simulink subsystem "tcp_trace_simscape_ref_subsys"  (R2022b)
settings: Solver=VariableStepAuto  StartTime=0.0  StopTime=10.0  RelTol=1e-3
undefined symbols (not defined in the file): param_vis
libraries: nesl_utility x300, sm_lib x200
(part 3 of 3)

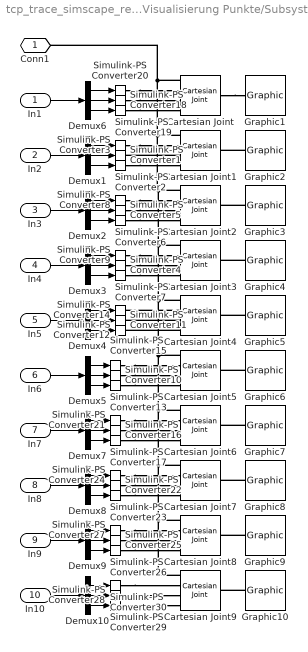
== system tcp_trace_simscape_ref_subsys/Visualisierung Punkte/Subsystem8 ==
  In1 : Inport
  In2 : Inport  Port=2
  In3 : Inport  Port=3
  In4 : Inport  Port=4
  In5 : Inport  Port=5
  In6 : Inport  Port=6
  In7 : Inport  Port=7
  In8 : Inport  Port=8
  In9 : Inport  Port=9
  In10 : Inport  Port=10
  Cartesian Joint{,1..9} (10 alike) : sm_lib/Joints/Cartesian Joint  JointMode=Normal  SenseConstraintForce=off  SenseConstraintForceX=off  SenseConstraintForceY=off  SenseConstraintForceZ=off  SenseConstraintTorque=off  SenseConstraintTorqueX=off  SenseConstraintTorqueY=off  SenseConstraintTorqueZ=off  SenseTotalForce=off  SenseTotalForceX=off  SenseTotalForceY=off  SenseTotalForceZ=off  SenseTotalTorque=off  SenseTotalTorqueX=off  SenseTotalTorqueY=off  SenseTotalTorqueZ=off  CompositeWrenchDir=FollowerOnBase  CompositeWrenchFrame=BaseFrame  PxEquilibriumPosition=0  PxEquilibriumPositionUnits=m  PxSpringStiffness=0  PxSpringStiffnessUnits=N/m  PxDampingCoefficient=0  PxDampingCoefficientUnits=N/(m/s)  PxTorqueActuationMode=ComputedTorque  PxMotionActuationMode=InputMotion  PxSensePosition=off  PxSenseVelocity=off  PxSenseAcceleration=off  PxSenseTorqueForce=off  PxSenseLowerLimitTorqueForce=off  PxSenseUpperLimitTorqueForce=off  PxLowerLimitSpecify=off  PxLowerLimitBound=-1  PxLowerLimitBoundUnits=m  PxLowerLimitStiffness=1e6  PxLowerLimitStiffnessUnits=N/m  PxLowerLimitDamping=1e3  PxLowerLimitDampingUnits=N/(m/s)  PxLowerLimitTransitionRegionWidth=1e-4  PxLowerLimitTransitionRegionWidthUnits=m  PxUpperLimitSpecify=off  PxUpperLimitBound=1  PxUpperLimitBoundUnits=m  PxUpperLimitStiffness=1e6  PxUpperLimitStiffnessUnits=N/m  PxUpperLimitDamping=1e3  PxUpperLimitDampingUnits=N/(m/s)  PxUpperLimitTransitionRegionWidth=1e-4  PxUpperLimitTransitionRegionWidthUnits=m  PxPositionTargetSpecify=off  PxPositionTargetPriority=High  PxPositionTargetValue=0  PxPositionTargetValueUnits=m  PxVelocityTargetSpecify=off  PxVelocityTargetPriority=High  PxVelocityTargetValue=0  PxVelocityTargetValueUnits=m/s  PyEquilibriumPosition=0  PyEquilibriumPositionUnits=m  PySpringStiffness=0  PySpringStiffnessUnits=N/m  PyDampingCoefficient=0  PyDampingCoefficientUnits=N/(m/s)  PyTorqueActuationMode=ComputedTorque  PyMotionActuationMode=InputMotion  PySensePosition=off  PySenseVelocity=off  PySenseAcceleration=off  PySenseTorqueForce=off  PySenseLowerLimitTorqueForce=off  PySenseUpperLimitTorqueForce=off  PyLowerLimitSpecify=off  PyLowerLimitBound=-1  PyLowerLimitBoundUnits=m  PyLowerLimitStiffness=1e6  PyLowerLimitStiffnessUnits=N/m  PyLowerLimitDamping=1e3  PyLowerLimitDampingUnits=N/(m/s)  PyLowerLimitTransitionRegionWidth=1e-4  PyLowerLimitTransitionRegionWidthUnits=m  PyUpperLimitSpecify=off  PyUpperLimitBound=1  PyUpperLimitBoundUnits=m  PyUpperLimitStiffness=1e6  PyUpperLimitStiffnessUnits=N/m  PyUpperLimitDamping=1e3  PyUpperLimitDampingUnits=N/(m/s)  PyUpperLimitTransitionRegionWidth=1e-4  PyUpperLimitTransitionRegionWidthUnits=m  PyPositionTargetSpecify=off  PyPositionTargetPriority=High  PyPositionTargetValue=0  PyPositionTargetValueUnits=m  PyVelocityTargetSpecify=off  PyVelocityTargetPriority=High  PyVelocityTargetValue=0  PyVelocityTargetValueUnits=m/s  PzEquilibriumPosition=0  PzEquilibriumPositionUnits=m  PzSpringStiffness=0  PzSpringStiffnessUnits=N/m  PzDampingCoefficient=0  PzDampingCoefficientUnits=N/(m/s)  PzTorqueActuationMode=ComputedTorque  PzMotionActuationMode=InputMotion  PzSensePosition=off  PzSenseVelocity=off  PzSenseAcceleration=off  PzSenseTorqueForce=off  PzSenseLowerLimitTorqueForce=off  PzSenseUpperLimitTorqueForce=off  PzLowerLimitSpecify=off  PzLowerLimitBound=-1  PzLowerLimitBoundUnits=m  PzLowerLimitStiffness=1e6  PzLowerLimitStiffnessUnits=N/m  PzLowerLimitDamping=1e3  PzLowerLimitDampingUnits=N/(m/s)  PzLowerLimitTransitionRegionWidth=1e-4  PzLowerLimitTransitionRegionWidthUnits=m  PzUpperLimitSpecify=off  PzUpperLimitBound=1  PzUpperLimitBoundUnits=m  PzUpperLimitStiffness=1e6  PzUpperLimitStiffnessUnits=N/m  PzUpperLimitDamping=1e3  PzUpperLimitDampingUnits=N/(m/s)  PzUpperLimitTransitionRegionWidth=1e-4  PzUpperLimitTransitionRegionWidthUnits=m  PzPositionTargetSpecify=off  PzPositionTargetPriority=High  PzPositionTargetValue=0  PzPositionTargetValueUnits=m  PzVelocityTargetSpecify=off  PzVelocityTargetPriority=High  PzVelocityTargetValue=0  PzVelocityTargetValueUnits=m/s
  Demux{1..10} (10 alike) : Demux  Outputs=3
  Graphic{1..10} (10 alike) : sm_lib/Body Elements/Graphic  GraphicType=Marker  MarkerShape=Sphere  MarkerSize=param_vis.vis_point.pix  GraphicVisPropType=SimpleVisualProperties  GraphicDiffuseColor=param_vis.vis_point.col  GraphicSpecularColor=[0.5 0.5 0.5 1.0]  GraphicAmbientColor=[0.15 0.15 0.15 1.0]  GraphicEmissiveColor=[0.0 0.0 0.0 1.0]  GraphicShininess=75  GraphicOpacity=param_vis.vis_point.opa
  Simulink-PS Converter{1..30} (30 alike) : nesl_utility/Simulink-PS Converter  PhysicalDomain=network_engine_domain  SubClassName=ps_input  LeftPortType=input  RightPortType=output  PseudoPeriodic=off  Frequencies=[]  NoiseDistribution=none  NoiseParameters=[]  Unit=1  AffineConversion=off  FilteringAndDerivatives=zero  SimscapeFilterOrder=2  InputFilterTimeConstant=0.001  UdotUserProvided=0
  Conn1 : PMIOPort  Side=Left
  wires:
  In7/1 -> Demux7/1
  In6/1 -> Demux5/1
  In10/1 -> Demux10/1
  In2/1 -> Demux1/1
  In5/1 -> Demux4/1
  In4/1 -> Demux3/1
  Demux6/3 -> Simulink-PS Converter19/1
  In3/1 -> Demux2/1
  In1/1 -> Demux6/1
  In9/1 -> Demux9/1
  In8/1 -> Demux8/1
  Demux6/1 -> Simulink-PS Converter20/1
  Demux6/2 -> Simulink-PS Converter18/1
  Demux1/1 -> Simulink-PS Converter3/1
  Demux4/2 -> Simulink-PS Converter11/1
  Demux4/1 -> Simulink-PS Converter14/1
  Demux4/3 -> Simulink-PS Converter12/1
  Demux1/2 -> Simulink-PS Converter1/1
  Demux1/3 -> Simulink-PS Converter2/1
  Demux2/1 -> Simulink-PS Converter8/1
  Demux2/2 -> Simulink-PS Converter5/1
  Demux2/3 -> Simulink-PS Converter6/1
  Demux3/3 -> Simulink-PS Converter7/1
  Demux3/1 -> Simulink-PS Converter9/1
  Demux3/2 -> Simulink-PS Converter4/1
  Demux5/1 -> Simulink-PS Converter15/1
  Demux5/2 -> Simulink-PS Converter10/1
  Demux5/3 -> Simulink-PS Converter13/1
  Demux7/1 -> Simulink-PS Converter21/1
  Demux7/2 -> Simulink-PS Converter16/1
  Demux7/3 -> Simulink-PS Converter17/1
  Demux8/1 -> Simulink-PS Converter24/1
  Demux8/2 -> Simulink-PS Converter22/1
  Demux8/3 -> Simulink-PS Converter23/1
  Demux9/1 -> Simulink-PS Converter27/1
  Demux9/2 -> Simulink-PS Converter25/1
  Demux9/3 -> Simulink-PS Converter26/1
  Demux10/1 -> Simulink-PS Converter30/1
  Demux10/2 -> Simulink-PS Converter28/1
  Demux10/3 -> Simulink-PS Converter29/1
  connections:
  Simulink-PS Converter19/RConn1 -- Cartesian Joint/LConn4
  Graphic4/RConn1 -- Cartesian Joint3/RConn1
  Cartesian Joint/RConn1 -- Graphic1/RConn1
  Graphic3/RConn1 -- Cartesian Joint2/RConn1
  Cartesian Joint8/LConn1 -- Cartesian Joint9/LConn1 -- Cartesian Joint7/LConn1 -- Cartesian Joint6/LConn1 -- Cartesian Joint5/LConn1 -- Cartesian Joint4/LConn1 -- Cartesian Joint3/LConn1 -- Cartesian Joint2/LConn1 -- Cartesian Joint1/LConn1 -- Cartesian Joint/LConn1 -- Conn1/RConn1
  Graphic7/RConn1 -- Cartesian Joint6/RConn1
  Graphic8/RConn1 -- Cartesian Joint7/RConn1
  Graphic6/RConn1 -- Cartesian Joint5/RConn1
  Graphic9/RConn1 -- Cartesian Joint8/RConn1
  Graphic2/RConn1 -- Cartesian Joint1/RConn1
  Graphic5/RConn1 -- Cartesian Joint4/RConn1
  Graphic10/RConn1 -- Cartesian Joint9/RConn1
  Simulink-PS Converter18/RConn1 -- Cartesian Joint/LConn3
  Simulink-PS Converter20/RConn1 -- Cartesian Joint/LConn2
  Simulink-PS Converter6/RConn1 -- Cartesian Joint2/LConn4
  Simulink-PS Converter8/RConn1 -- Cartesian Joint2/LConn2
  Simulink-PS Converter5/RConn1 -- Cartesian Joint2/LConn3
  Cartesian Joint4/LConn4 -- Simulink-PS Converter12/RConn1
  Cartesian Joint4/LConn2 -- Simulink-PS Converter14/RConn1
  Cartesian Joint4/LConn3 -- Simulink-PS Converter11/RConn1
  Simulink-PS Converter3/RConn1 -- Cartesian Joint1/LConn2
  Cartesian Joint1/LConn3 -- Simulink-PS Converter1/RConn1
  Simulink-PS Converter2/RConn1 -- Cartesian Joint1/LConn4
  Simulink-PS Converter15/RConn1 -- Cartesian Joint5/LConn2
  Simulink-PS Converter10/RConn1 -- Cartesian Joint5/LConn3
  Simulink-PS Converter13/RConn1 -- Cartesian Joint5/LConn4
  Simulink-PS Converter21/RConn1 -- Cartesian Joint6/LConn2
  Simulink-PS Converter16/RConn1 -- Cartesian Joint6/LConn3
  Simulink-PS Converter17/RConn1 -- Cartesian Joint6/LConn4
  Simulink-PS Converter24/RConn1 -- Cartesian Joint7/LConn2
  Simulink-PS Converter22/RConn1 -- Cartesian Joint7/LConn3
  Simulink-PS Converter23/RConn1 -- Cartesian Joint7/LConn4
  Simulink-PS Converter27/RConn1 -- Cartesian Joint8/LConn2
  Simulink-PS Converter25/RConn1 -- Cartesian Joint8/LConn3
  Simulink-PS Converter26/RConn1 -- Cartesian Joint8/LConn4
  Simulink-PS Converter30/RConn1 -- Cartesian Joint9/LConn2
  Simulink-PS Converter28/RConn1 -- Cartesian Joint9/LConn3
  Simulink-PS Converter29/RConn1 -- Cartesian Joint9/LConn4
  Simulink-PS Converter9/RConn1 -- Cartesian Joint3/LConn2
  Simulink-PS Converter4/RConn1 -- Cartesian Joint3/LConn3
  Simulink-PS Converter7/RConn1 -- Cartesian Joint3/LConn4

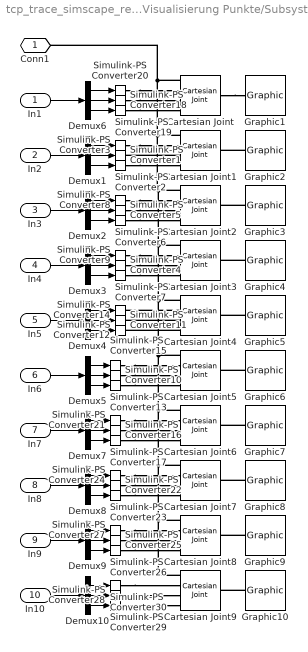
== system tcp_trace_simscape_ref_subsys/Visualisierung Punkte/Subsystem9 ==
  In1 : Inport
  In2 : Inport  Port=2
  In3 : Inport  Port=3
  In4 : Inport  Port=4
  In5 : Inport  Port=5
  In6 : Inport  Port=6
  In7 : Inport  Port=7
  In8 : Inport  Port=8
  In9 : Inport  Port=9
  In10 : Inport  Port=10
  Cartesian Joint{,1..9} (10 alike) : sm_lib/Joints/Cartesian Joint  JointMode=Normal  SenseConstraintForce=off  SenseConstraintForceX=off  SenseConstraintForceY=off  SenseConstraintForceZ=off  SenseConstraintTorque=off  SenseConstraintTorqueX=off  SenseConstraintTorqueY=off  SenseConstraintTorqueZ=off  SenseTotalForce=off  SenseTotalForceX=off  SenseTotalForceY=off  SenseTotalForceZ=off  SenseTotalTorque=off  SenseTotalTorqueX=off  SenseTotalTorqueY=off  SenseTotalTorqueZ=off  CompositeWrenchDir=FollowerOnBase  CompositeWrenchFrame=BaseFrame  PxEquilibriumPosition=0  PxEquilibriumPositionUnits=m  PxSpringStiffness=0  PxSpringStiffnessUnits=N/m  PxDampingCoefficient=0  PxDampingCoefficientUnits=N/(m/s)  PxTorqueActuationMode=ComputedTorque  PxMotionActuationMode=InputMotion  PxSensePosition=off  PxSenseVelocity=off  PxSenseAcceleration=off  PxSenseTorqueForce=off  PxSenseLowerLimitTorqueForce=off  PxSenseUpperLimitTorqueForce=off  PxLowerLimitSpecify=off  PxLowerLimitBound=-1  PxLowerLimitBoundUnits=m  PxLowerLimitStiffness=1e6  PxLowerLimitStiffnessUnits=N/m  PxLowerLimitDamping=1e3  PxLowerLimitDampingUnits=N/(m/s)  PxLowerLimitTransitionRegionWidth=1e-4  PxLowerLimitTransitionRegionWidthUnits=m  PxUpperLimitSpecify=off  PxUpperLimitBound=1  PxUpperLimitBoundUnits=m  PxUpperLimitStiffness=1e6  PxUpperLimitStiffnessUnits=N/m  PxUpperLimitDamping=1e3  PxUpperLimitDampingUnits=N/(m/s)  PxUpperLimitTransitionRegionWidth=1e-4  PxUpperLimitTransitionRegionWidthUnits=m  PxPositionTargetSpecify=off  PxPositionTargetPriority=High  PxPositionTargetValue=0  PxPositionTargetValueUnits=m  PxVelocityTargetSpecify=off  PxVelocityTargetPriority=High  PxVelocityTargetValue=0  PxVelocityTargetValueUnits=m/s  PyEquilibriumPosition=0  PyEquilibriumPositionUnits=m  PySpringStiffness=0  PySpringStiffnessUnits=N/m  PyDampingCoefficient=0  PyDampingCoefficientUnits=N/(m/s)  PyTorqueActuationMode=ComputedTorque  PyMotionActuationMode=InputMotion  PySensePosition=off  PySenseVelocity=off  PySenseAcceleration=off  PySenseTorqueForce=off  PySenseLowerLimitTorqueForce=off  PySenseUpperLimitTorqueForce=off  PyLowerLimitSpecify=off  PyLowerLimitBound=-1  PyLowerLimitBoundUnits=m  PyLowerLimitStiffness=1e6  PyLowerLimitStiffnessUnits=N/m  PyLowerLimitDamping=1e3  PyLowerLimitDampingUnits=N/(m/s)  PyLowerLimitTransitionRegionWidth=1e-4  PyLowerLimitTransitionRegionWidthUnits=m  PyUpperLimitSpecify=off  PyUpperLimitBound=1  PyUpperLimitBoundUnits=m  PyUpperLimitStiffness=1e6  PyUpperLimitStiffnessUnits=N/m  PyUpperLimitDamping=1e3  PyUpperLimitDampingUnits=N/(m/s)  PyUpperLimitTransitionRegionWidth=1e-4  PyUpperLimitTransitionRegionWidthUnits=m  PyPositionTargetSpecify=off  PyPositionTargetPriority=High  PyPositionTargetValue=0  PyPositionTargetValueUnits=m  PyVelocityTargetSpecify=off  PyVelocityTargetPriority=High  PyVelocityTargetValue=0  PyVelocityTargetValueUnits=m/s  PzEquilibriumPosition=0  PzEquilibriumPositionUnits=m  PzSpringStiffness=0  PzSpringStiffnessUnits=N/m  PzDampingCoefficient=0  PzDampingCoefficientUnits=N/(m/s)  PzTorqueActuationMode=ComputedTorque  PzMotionActuationMode=InputMotion  PzSensePosition=off  PzSenseVelocity=off  PzSenseAcceleration=off  PzSenseTorqueForce=off  PzSenseLowerLimitTorqueForce=off  PzSenseUpperLimitTorqueForce=off  PzLowerLimitSpecify=off  PzLowerLimitBound=-1  PzLowerLimitBoundUnits=m  PzLowerLimitStiffness=1e6  PzLowerLimitStiffnessUnits=N/m  PzLowerLimitDamping=1e3  PzLowerLimitDampingUnits=N/(m/s)  PzLowerLimitTransitionRegionWidth=1e-4  PzLowerLimitTransitionRegionWidthUnits=m  PzUpperLimitSpecify=off  PzUpperLimitBound=1  PzUpperLimitBoundUnits=m  PzUpperLimitStiffness=1e6  PzUpperLimitStiffnessUnits=N/m  PzUpperLimitDamping=1e3  PzUpperLimitDampingUnits=N/(m/s)  PzUpperLimitTransitionRegionWidth=1e-4  PzUpperLimitTransitionRegionWidthUnits=m  PzPositionTargetSpecify=off  PzPositionTargetPriority=High  PzPositionTargetValue=0  PzPositionTargetValueUnits=m  PzVelocityTargetSpecify=off  PzVelocityTargetPriority=High  PzVelocityTargetValue=0  PzVelocityTargetValueUnits=m/s
  Demux{1..10} (10 alike) : Demux  Outputs=3
  Graphic{1..10} (10 alike) : sm_lib/Body Elements/Graphic  GraphicType=Marker  MarkerShape=Sphere  MarkerSize=param_vis.vis_point.pix  GraphicVisPropType=SimpleVisualProperties  GraphicDiffuseColor=param_vis.vis_point.col  GraphicSpecularColor=[0.5 0.5 0.5 1.0]  GraphicAmbientColor=[0.15 0.15 0.15 1.0]  GraphicEmissiveColor=[0.0 0.0 0.0 1.0]  GraphicShininess=75  GraphicOpacity=param_vis.vis_point.opa
  Simulink-PS Converter{1..30} (30 alike) : nesl_utility/Simulink-PS Converter  PhysicalDomain=network_engine_domain  SubClassName=ps_input  LeftPortType=input  RightPortType=output  PseudoPeriodic=off  Frequencies=[]  NoiseDistribution=none  NoiseParameters=[]  Unit=1  AffineConversion=off  FilteringAndDerivatives=zero  SimscapeFilterOrder=2  InputFilterTimeConstant=0.001  UdotUserProvided=0
  Conn1 : PMIOPort  Side=Left
  wires:
  Demux10/3 -> Simulink-PS Converter29/1
  Demux10/2 -> Simulink-PS Converter28/1
  Demux10/1 -> Simulink-PS Converter30/1
  Demux9/3 -> Simulink-PS Converter26/1
  Demux9/2 -> Simulink-PS Converter25/1
  Demux9/1 -> Simulink-PS Converter27/1
  Demux8/3 -> Simulink-PS Converter23/1
  Demux8/2 -> Simulink-PS Converter22/1
  Demux8/1 -> Simulink-PS Converter24/1
  Demux7/3 -> Simulink-PS Converter17/1
  Demux7/2 -> Simulink-PS Converter16/1
  Demux7/1 -> Simulink-PS Converter21/1
  Demux5/3 -> Simulink-PS Converter13/1
  Demux5/2 -> Simulink-PS Converter10/1
  Demux5/1 -> Simulink-PS Converter15/1
  Demux3/2 -> Simulink-PS Converter4/1
  Demux3/1 -> Simulink-PS Converter9/1
  Demux3/3 -> Simulink-PS Converter7/1
  Demux2/3 -> Simulink-PS Converter6/1
  Demux2/2 -> Simulink-PS Converter5/1
  Demux2/1 -> Simulink-PS Converter8/1
  Demux1/3 -> Simulink-PS Converter2/1
  Demux1/2 -> Simulink-PS Converter1/1
  Demux4/3 -> Simulink-PS Converter12/1
  Demux4/1 -> Simulink-PS Converter14/1
  Demux4/2 -> Simulink-PS Converter11/1
  Demux1/1 -> Simulink-PS Converter3/1
  Demux6/2 -> Simulink-PS Converter18/1
  Demux6/1 -> Simulink-PS Converter20/1
  In8/1 -> Demux8/1
  In9/1 -> Demux9/1
  In1/1 -> Demux6/1
  In3/1 -> Demux2/1
  Demux6/3 -> Simulink-PS Converter19/1
  In4/1 -> Demux3/1
  In5/1 -> Demux4/1
  In2/1 -> Demux1/1
  In10/1 -> Demux10/1
  In6/1 -> Demux5/1
  In7/1 -> Demux7/1
  connections:
  Simulink-PS Converter7/RConn1 -- Cartesian Joint3/LConn4
  Simulink-PS Converter4/RConn1 -- Cartesian Joint3/LConn3
  Simulink-PS Converter9/RConn1 -- Cartesian Joint3/LConn2
  Simulink-PS Converter29/RConn1 -- Cartesian Joint9/LConn4
  Simulink-PS Converter28/RConn1 -- Cartesian Joint9/LConn3
  Simulink-PS Converter30/RConn1 -- Cartesian Joint9/LConn2
  Simulink-PS Converter26/RConn1 -- Cartesian Joint8/LConn4
  Simulink-PS Converter25/RConn1 -- Cartesian Joint8/LConn3
  Simulink-PS Converter27/RConn1 -- Cartesian Joint8/LConn2
  Simulink-PS Converter23/RConn1 -- Cartesian Joint7/LConn4
  Simulink-PS Converter22/RConn1 -- Cartesian Joint7/LConn3
  Simulink-PS Converter24/RConn1 -- Cartesian Joint7/LConn2
  Simulink-PS Converter17/RConn1 -- Cartesian Joint6/LConn4
  Simulink-PS Converter16/RConn1 -- Cartesian Joint6/LConn3
  Simulink-PS Converter21/RConn1 -- Cartesian Joint6/LConn2
  Simulink-PS Converter13/RConn1 -- Cartesian Joint5/LConn4
  Simulink-PS Converter10/RConn1 -- Cartesian Joint5/LConn3
  Simulink-PS Converter15/RConn1 -- Cartesian Joint5/LConn2
  Simulink-PS Converter2/RConn1 -- Cartesian Joint1/LConn4
  Cartesian Joint1/LConn3 -- Simulink-PS Converter1/RConn1
  Simulink-PS Converter3/RConn1 -- Cartesian Joint1/LConn2
  Cartesian Joint4/LConn3 -- Simulink-PS Converter11/RConn1
  Cartesian Joint4/LConn2 -- Simulink-PS Converter14/RConn1
  Cartesian Joint4/LConn4 -- Simulink-PS Converter12/RConn1
  Simulink-PS Converter5/RConn1 -- Cartesian Joint2/LConn3
  Simulink-PS Converter8/RConn1 -- Cartesian Joint2/LConn2
  Simulink-PS Converter6/RConn1 -- Cartesian Joint2/LConn4
  Simulink-PS Converter20/RConn1 -- Cartesian Joint/LConn2
  Simulink-PS Converter18/RConn1 -- Cartesian Joint/LConn3
  Graphic10/RConn1 -- Cartesian Joint9/RConn1
  Graphic5/RConn1 -- Cartesian Joint4/RConn1
  Graphic2/RConn1 -- Cartesian Joint1/RConn1
  Graphic9/RConn1 -- Cartesian Joint8/RConn1
  Graphic6/RConn1 -- Cartesian Joint5/RConn1
  Graphic8/RConn1 -- Cartesian Joint7/RConn1
  Graphic7/RConn1 -- Cartesian Joint6/RConn1
  Conn1/RConn1 -- Cartesian Joint/LConn1 -- Cartesian Joint1/LConn1 -- Cartesian Joint2/LConn1 -- Cartesian Joint3/LConn1 -- Cartesian Joint4/LConn1 -- Cartesian Joint5/LConn1 -- Cartesian Joint6/LConn1 -- Cartesian Joint7/LConn1 -- Cartesian Joint9/LConn1 -- Cartesian Joint8/LConn1
  Graphic3/RConn1 -- Cartesian Joint2/RConn1
  Cartesian Joint/RConn1 -- Graphic1/RConn1
  Graphic4/RConn1 -- Cartesian Joint3/RConn1
  Simulink-PS Converter19/RConn1 -- Cartesian Joint/LConn4

== matlab function tcp_trace_simscape_ref_subsys/MATLAB Function ==
  settings: updateMethod=DISCRETE  sampleTime=param_global.Ta
  data: robot_model input; p1 output; p2 output; p3 output; p4 output; p5 output; p6 output; p7 output; p8 output; p9 output; p10 output; p11 output; p12 output; p13 output; p14 output; p15 output; p16 output; p17 output; p18 output; p19 output; p20 output; p21 output; p22 output; p23 output; p24 output; p25 output; p26 output; p27 output; p28 output; p29 output; p30 output; p31 output; p32 output; p33 output; p34 output; p35 output; p36 output; p37 output; p38 output; p39 output; p40 output; p41 output; p42 output; p43 output; p44 output; p45 output; p46 output; p47 output; p48 output; p49 output; p50 output; start input; delta input; p51 output; p52 output; p53 output; p54 output; p55 output; p56 output; p57 output; p58 output; p59 output; p60 output; p61 output; p62 output; p63 output; p64 output; p65 output; p66 output; p67 output; p68 output; p69 output; p70 output; p71 output; p72 output; p73 output; p74 output; p75 output; p76 output; p77 output; p78 output; p79 output; p80 output; p81 output; p82 output; p83 output; p84 output; p85 output; p86 output; p87 output; p88 output; p89 output; p90 output; p91 output; p92 output; p93 output; p94 output; p95 output; p96 output; p97 output; p98 output; p99 output; p100 output
function [p1,p2,p3,p4,p5,p6,p7,p8,p9,p10,p11,p12,p13,p14,p15,p16,p17,p18,p19,p20,p21,p22,p23,p24,p25,p26,p27,p28,p29,p30,p31,p32,p33,p34,p35,p36,p37,p38,p39,p40,p41,p42,p43,p44,p45,p46,p47,p48,p49,p50,p51,p52,p53,p54,p55,p56,p57,p58,p59,p60,p61,p62,p63,p64,p65,p66,p67,p68,p69,p70,p71,p72,p73,p74,p75,p76,p77,p78,p79,p80,p81,p82,p83,p84,p85,p86,p87,p88,p89,p90,p91,p92,p93,p94,p95,p96,p97,p98,p99,p100] = fcn(robot_model, start, delta)
persistent i t1 t2 t3 t4 t5 t6 t7 t8 t9 t10 t11 t12 t13 t14 t15 t16 t17 t18 t19 t20 t21 t22 t23 t24 t25 t26 t27 t28 t29 t30 t31 t32 t33 t34 t35 t36 t37 t38 t39 t40 t41 t42 t43 t44 t45 t46 t47 t48 t49 t50 t51 t52 t53 t54 t55 t56 t57 t58 t59 t60 t61 t62 t63 t64 t65 t66 t67 t68 t69 t70 t71 t72 t73 t74 t75 t76 t77 t78 t79 t80 t81 t82 t83 t84 t85 t86 t87 t88 t89 t90 t91 t92 t93 t94 t95 t96 t97 t98 t99 t100
if isempty(t1)
    i = 1;
    t1 = robot_model.H(1:3,4);
    t2 = t1;
    t3 = t1;
    t4 = t1;
    t5 = t1;
    t6 = t1;
    t7 = t1;
    t8 = t1;
    t9 = t1;
    t10 = t1;
    t11 = t1;
    t12 = t1;
    t13 = t1;
    t14 = t1;
    t15 = t1;
    t16 = t1;
    t17 = t1;
    t18 = t1;
    t19 = t1;
    t20 = t1;
    t21 = t1;
    t22 = t1;
    t23 = t1;
    t24 = t1;
    t25 = t1;
    t26 = t1;
    t27 = t1;
    t28 = t1;
    t29 = t1;
    t30 = t1;
    t31 = t1;
    t32 = t1;
    t33 = t1;
    t34 = t1;
    t35 = t1;
    t36 = t1;
    t37 = t1;
    t38 = t1;
    t39 = t1;
    t40 = t1;
    t41 = t1;
    t42 = t1;
    t43 = t1;
    t44 = t1;
    t45 = t1;
    t46 = t1;
    t47 = t1;
    t48 = t1;
    t49 = t1;
    t50 = t1;
    t51 = t1;
    t52 = t1;
    t53 = t1;
    t54 = t1;
    t55 = t1;
    t56 = t1;
    t57 = t1;
    t58 = t1;
    t59 = t1;
    t60 = t1;
    t61 = t1;
    t62 = t1;
    t63 = t1;
    t64 = t1;
    t65 = t1;
    t66 = t1;
    t67 = t1;
    t68 = t1;
    t69 = t1;
    t70 = t1;
    t71 = t1;
    t72 = t1;
    t73 = t1;
    t74 = t1;
    t75 = t1;
    t76 = t1;
    t77 = t1;
    t78 = t1;
    t79 = t1;
    t80 = t1;
    t81 = t1;
    t82 = t1;
    t83 = t1;
    t84 = t1;
    t85 = t1;
    t86 = t1;
    t87 = t1;
    t88 = t1;
    t89 = t1;
    t90 = t1;
    t91 = t1;
    t92 = t1;
    t93 = t1;
    t94 = t1;
    t95 = t1;
    t96 = t1;
    t97 = t1;
    t98 = t1;
    t99 = t1;
    t100 = t1;
    
end

switch i
    case start
        t1 = robot_model.H(1:3,4);
    case start+delta*1
        t2 = robot_model.H(1:3,4);
    case start+delta*2
        t3 = robot_model.H(1:3,4);
    case start+delta*3
        t4 = robot_model.H(1:3,4);
    case start+delta*4
        t5 = robot_model.H(1:3,4);
    case start+delta*5
        t6 = robot_model.H(1:3,4);
    case start+delta*6
        t7 = robot_model.H(1:3,4);
    case start+delta*7
        t8 = robot_model.H(1:3,4);
    case start+delta*8
        t9 = robot_model.H(1:3,4);
    case start+delta*9
        t10 = robot_model.H(1:3,4);
    case start+delta*10
        t11 = robot_model.H(1:3,4);
    case start+delta*11
        t12 = robot_model.H(1:3,4);
    case start+delta*12
        t13 = robot_model.H(1:3,4);
    case start+delta*13
        t14 = robot_model.H(1:3,4);
    case start+delta*14
        t15 = robot_model.H(1:3,4);
    case start+delta*15
        t16 = robot_model.H(1:3,4);
    case start+delta*16
        t17 = robot_model.H(1:3,4);
    case start+delta*17
        t18 = robot_model.H(1:3,4);
    case start+delta*18
        t19 = robot_model.H(1:3,4);
    case start+delta*19
        t20 = robot_model.H(1:3,4);
    case start+delta*20
        t21 = robot_model.H(1:3,4);
    case start+delta*21
        t22 = robot_model.H(1:3,4);
    case start+delta*22
        t23 = robot_model.H(1:3,4);
    case start+delta*23
        t24 = robot_model.H(1:3,4);
    case start+delta*24
        t25 = robot_model.H(1:3,4);
    case start+delta*25
        t26 = robot_model.H(1:3,4);
    case start+delta*26
        t27 = robot_model.H(1:3,4);
    case start+delta*27
        t28 = robot_model.H(1:3,4);
    case start+delta*28
        t29 = robot_model.H(1:3,4);
    case start+delta*29
        t30 = robot_model.H(1:3,4);
    case start+delta*30
        t31 = robot_model.H(1:3,4);
    case start+delta*31
        t32 = robot_model.H(1:3,4);
    case start+delta*32
        t33 = robot_model.H(1:3,4);
    case start+delta*33
        t34 = robot_model.H(1:3,4);
    case start+delta*34
        t35 = robot_model.H(1:3,4);
    case start+delta*35
        t36 = robot_model.H(1:3,4);
    case start+delta*36
        t37 = robot_model.H(1:3,4);
    case start+delta*37
        t38 = robot_model.H(1:3,4);
    case start+delta*38
        t39 = robot_model.H(1:3,4);
    case start+delta*39
        t40 = robot_model.H(1:3,4);
    case start+delta*40
        t41 = robot_model.H(1:3,4);
    case start+delta*41
        t42 = robot_model.H(1:3,4);
    case start+delta*42
        t43 = robot_model.H(1:3,4);
    case start+delta*43
        t44 = robot_model.H(1:3,4);
    case start+delta*44
        t45 = robot_model.H(1:3,4);
    case start+delta*45
        t46 = robot_model.H(1:3,4);
    case start+delta*46
        t47 = robot_model.H(1:3,4);
    case start+delta*47
        t48 = robot_model.H(1:3,4);
    case start+delta*48
        t49 = robot_model.H(1:3,4);
    case start+delta*49
        t50 = robot_model.H(1:3,4);
    case start+delta*50
        t51 = robot_model.H(1:3,4);
    case start+delta*51
        t52 = robot_model.H(1:3,4);
    case start+delta*52
        t53 = robot_model.H(1:3,4);
    case start+delta*53
        t54 = robot_model.H(1:3,4);
    case start+delta*54
        t55 = robot_model.H(1:3,4);
    case start+delta*55
        t56 = robot_model.H(1:3,4);
    case start+delta*56
        t57 = robot_model.H(1:3,4);
    case start+delta*57
        t58 = robot_model.H(1:3,4);
    case start+delta*58
        t59 = robot_model.H(1:3,4);
    case start+delta*59
        t60 = robot_model.H(1:3,4);
    case start+delta*60
        t61 = robot_model.H(1:3,4);
    case start+delta*61
        t62 = robot_model.H(1:3,4);
    case start+delta*62
        t63 = robot_model.H(1:3,4);
    case start+delta*63
        t64 = robot_model.H(1:3,4);
    case start+delta*64
        t65 = robot_model.H(1:3,4);
    case start+delta*65
        t66 = robot_model.H(1:3,4);
    case start+delta*66
        t67 = robot_model.H(1:3,4);
    case start+delta*67
        t68 = robot_model.H(1:3,4);
    case start+delta*68
        t69 = robot_model.H(1:3,4);
    case start+delta*69
        t70 = robot_model.H(1:3,4);
    case start+delta*70
        t71 = robot_model.H(1:3,4);
    case start+delta*71
        t72 = robot_model.H(1:3,4);
    case start+delta*72
        t73 = robot_model.H(1:3,4);
    case start+delta*73
        t74 = robot_model.H(1:3,4);
    case start+delta*74
        t75 = robot_model.H(1:3,4);
    case start+delta*75
        t76 = robot_model.H(1:3,4);
    case start+delta*76
        t77 = robot_model.H(1:3,4);
    case start+delta*77
        t78 = robot_model.H(1:3,4);
    case start+delta*78
        t79 = robot_model.H(1:3,4);
    case start+delta*79
        t80 = robot_model.H(1:3,4);
    case start+delta*80
        t81 = robot_model.H(1:3,4);
    case start+delta*81
        t82 = robot_model.H(1:3,4);
    case start+delta*82
        t83 = robot_model.H(1:3,4);
    case start+delta*83
        t84 = robot_model.H(1:3,4);
    case start+delta*84
        t85 = robot_model.H(1:3,4);
    case start+delta*85
        t86 = robot_model.H(1:3,4);
    case start+delta*86
        t87 = robot_model.H(1:3,4);
    case start+delta*87
        t88 = robot_model.H(1:3,4);
    case start+delta*88
        t89 = robot_model.H(1:3,4);
    case start+delta*89
        t90 = robot_model.H(1:3,4);
    case start+delta*90
        t91 = robot_model.H(1:3,4);
    case start+delta*91
        t92 = robot_model.H(1:3,4);
    case start+delta*92
        t93 = robot_model.H(1:3,4);
    case start+delta*93
        t94 = robot_model.H(1:3,4);
    case start+delta*94
        t95 = robot_model.H(1:3,4);
    case start+delta*95
        t96 = robot_model.H(1:3,4);
    case start+delta*96
        t97 = robot_model.H(1:3,4);
    case start+delta*97
        t98 = robot_model.H(1:3,4);
    case start+delta*98
        t99 = robot_model.H(1:3,4);
    case start+delta*99
        t100 = robot_model.H(1:3,4);
end

i = i+1;
p1 = t1;
p2 = t2;
p3 = t3;
p4 = t4;
p5 = t5;
p6 = t6;
p7 = t7;
p8 = t8;
p9 = t9;
p10 = t10;
p11 = t11;
p12 = t12;
p13 = t13;
p14 = t14;
p15 = t15;
p16 = t16;
p17 = t17;
p18 = t18;
p19 = t19;
p20 = t20;
p21 = t21;
p22 = t22;
p23 = t23;
p24 = t24;
p25 = t25;
p26 = t26;
p27 = t27;
p28 = t28;
p29 = t29;
p30 = t30;
p31 = t31;
p32 = t32;
p33 = t33;
p34 = t34;
p35 = t35;
p36 = t36;
p37 = t37;
p38 = t38;
p39 = t39;
p40 = t40;
p41 = t41;
p42 = t42;
p43 = t43;
p44 = t44;
p45 = t45;
p46 = t46;
p47 = t47;
p48 = t48;
p49 = t49;
p50 = t50;
p51 = t51;
p52 = t52;
p53 = t53;
p54 = t54;
p55 = t55;
p56 = t56;
p57 = t57;
p58 = t58;
p59 = t59;
p60 = t60;
p61 = t61;
p62 = t62;
p63 = t63;
p64 = t64;
p65 = t65;
p66 = t66;
p67 = t67;
p68 = t68;
p69 = t69;
p70 = t70;
p71 = t71;
p72 = t72;
p73 = t73;
p74 = t74;
p75 = t75;
p76 = t76;
p77 = t77;
p78 = t78;
p79 = t79;
p80 = t80;
p81 = t81;
p82 = t82;
p83 = t83;
p84 = t84;
p85 = t85;
p86 = t86;
p87 = t87;
p88 = t88;
p89 = t89;
p90 = t90;
p91 = t91;
p92 = t92;
p93 = t93;
p94 = t94;
p95 = t95;
p96 = t96;
p97 = t97;
p98 = t98;
p99 = t99;
p100 = t100;
